simulink library "Energy_converter_Electrical_to_Mechanical"  (R2016a)
settings: Solver=ode1  StartTime=0.0  StopTime=Inf  FixedStep=0.001  RelTol=1e-3
undefined symbols (not defined in the file): API1dcac_efficiency, API2dcac_efficiency, API3dcac_efficiency, aux_power_state, AWR_InvStError, dat, DiscIntNeverNeededParam, EDCU_p_RefTqeMOT, emot_AcCmprFront_inertia, emot_AcCmprFront_nTab_3rdD, emot_AcCmprFront_pwrAC, emot_AcCmprFront_Tau, emot_AcCmprFront_trqTab_2ndD, emot_AcCmprFront_vltTab_1stD, emot_AcCmprRear_inertia, emot_AcCmprRear_nTab_3rdD, emot_AcCmprRear_pwrAC, emot_AcCmprRear_Tau, emot_AcCmprRear_trqTab_2ndD, emot_AcCmprRear_vltTab_1stD, emot_AirCmpr_inertia, emot_AirCmpr_nTab_3rdD, emot_AirCmpr_pwrAC, emot_AirCmpr_Tau, emot_AirCmpr_trqTab_2ndD, emot_AirCmpr_vltTab_1stD, emot_aircomp_power, emot_Cth_rotor, emot_Cth_stator, emot_dtrqEmotNeg, emot_dtrqEmotPtv, emot_inv_pwracTab_1st, emot_inv_pwrDC, emot_inv_pwrLoss, emot_inv_VrmsTab_2nd, emot_j, emot_mot_pwrLoss, emot_nTab_1stD, emot_pwrEtaTab_nRow, emot_pwrEtaTab_pwrTab, emot_pwrEtaTab_trqClm, emot_Rth_rotor_oil, emot_Rth_stator_oil, emot_Rth_stator_rotor, emot_tractiongroup, emot_Trotor_init, emot_trqMaxRow, emot_trqMinRow, emot_Tstator_init, emot_vltTab_3rdD, FirstDrivenAxleNoOfEmot, inv_Cth_cooling_plate, inv_Cth_diode, inv_Cth_IGBT, inv_n_IGBT_per_Switch, inv_Rth_cooling_plate_coolant, inv_Rth_PS_cooling_plate, inv_Tplate_init, inv_Tpowerstack_init, midAxleNoOfEmot ... (+6)
libraries: Electrical_converter x12, Energy_converter_Electrical_to_Mechanical x12, simulink x7
(part 6 of 8)

== system Energy_converter_Electrical_to_Mechanical/e-Motor/Thermic_Model_PMSM_slot2 ==
  P_WasteHeat_Rotor : Inport
  P_WasteHeat_Stator : Inport  Port=2
  T_Oil : Inport  Port=3
  T_Stator : Inport  Port=4
  T_Rotor : Inport  Port=5
  Add : Sum
  Add1 : Sum  Inputs=-+-
  Add2 : Sum  Inputs=++-
  C_Rotor : Subsystem
  C_Stator : Subsystem
  K2degC : Subsystem
  K2degC1 : Subsystem
  R_RotorOil : Subsystem
  R_StatorOil : Subsystem
  R_StatorRotor : Subsystem
  degC2K : Subsystem
  degC2K1 : Subsystem
  degC2K2 : Subsystem
  HeatFlow_eMotor_Oil : Outport
  T_Stator_new : Outport  Port=2
  T_Rotor_new : Outport  Port=3
  wires:
  C_Stator/1(T_new) -> K2degC/1(In1)
  C_Rotor/1(T_new) -> K2degC1/1(In1)
  Add/1 -> HeatFlow_eMotor_Oil/1
  R_StatorOil/1(dQ) -> Add1/1, Add/2
  [A] -> Add/1
  T_Stator/1 -> degC2K1/1(In1)
  P_WasteHeat_Stator/1 -> Add1/2
  Add1/1 -> C_Stator/1(P_Heat_eff)
  R_StatorRotor/1(dQ) -> Add2/1, Add1/3
  T_Rotor/1 -> degC2K2/1(In1)
  R_RotorOil/1(dQ) -> [A], Add2/3
  Add2/1 -> C_Rotor/1(P_Heat_eff)
  P_WasteHeat_Rotor/1 -> Add2/2
  K2degC/1(Out1) -> T_Stator_new/1
  K2degC1/1(Out1) -> T_Rotor_new/1
  T_Oil/1 -> degC2K/1(In1)  "T_Oil"
  degC2K/1(Out1) -> [B], R_StatorOil/1(T_Oil)
  degC2K1/1(Out1) -> R_StatorRotor/1(T_Stator), C_Stator/2(T), R_StatorOil/2(T_Stator)
  degC2K2/1(Out1) -> R_RotorOil/1(T_Rotor), C_Rotor/2(T), R_StatorRotor/2(T_Rotor)
  [B] -> R_RotorOil/2(T_Oil)

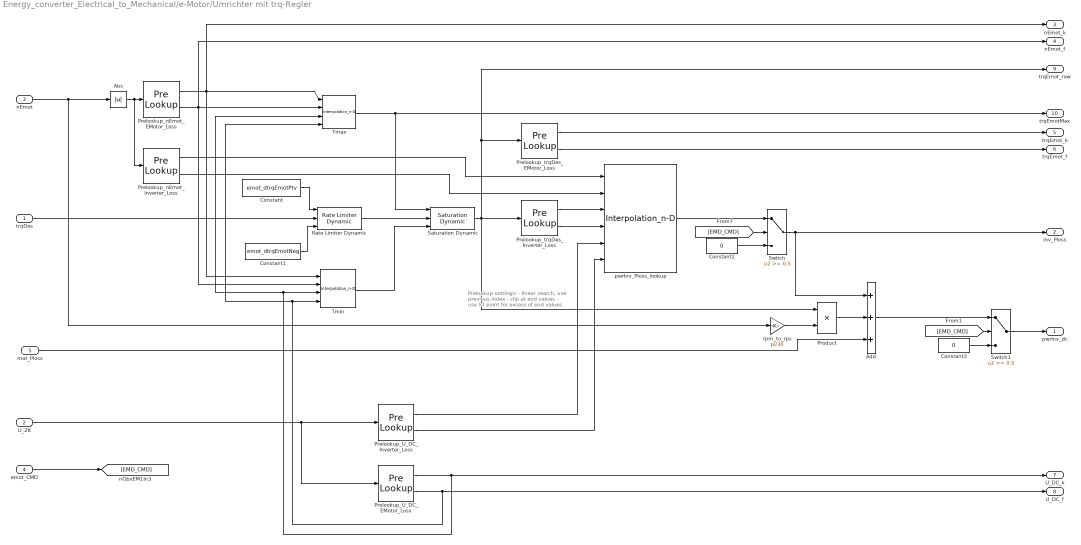
== system Energy_converter_Electrical_to_Mechanical/e-Motor/Umrichter mit trq-Regler ==
  note: Prelookup settings:
      | - linear search, use previous index
      | - clip at end values
      | - use lst point for
      | excess of end values
  trqDes : Inport
  U_ZK : Inport  Port=2
  nEmot : Inport  Port=3
  emot_CMD : Inport  Port=4
  mot_Ploss : Inport  Port=5
  Abs : Abs
  Add : Sum  Inputs=+++
  Constant : Constant  Value=emot_dtrqEmotPtv
  Constant1 : Constant  Value=emot_dtrqEmotNeg
  Constant2 : Constant  Value=0
  Constant3 : Constant  Value=0
  Prelookup_U_DC_EMotor_Loss : PreLookup  BreakpointsData=emot_vltTab_3rdD  IndexSearchMethod=Linear search  BeginIndexSearchUsingPreviousIndexResult=on  UseLastBreakpoint=on
  Prelookup_U_DC_Inverter_Loss : PreLookup  BreakpointsData=inv_vltTab_3rdD  IndexSearchMethod=Linear search  BeginIndexSearchUsingPreviousIndexResult=on  UseLastBreakpoint=on
  Prelookup_nEmot_EMotor_Loss : PreLookup  BreakpointsData=emot_nTab_1stD  IndexSearchMethod=Linear search  BeginIndexSearchUsingPreviousIndexResult=on  UseLastBreakpoint=on
  Prelookup_nEmot_Inverter_Loss : PreLookup  BreakpointsData=inv_nTab_1stD  IndexSearchMethod=Linear search  BeginIndexSearchUsingPreviousIndexResult=on  UseLastBreakpoint=on
  Prelookup_trqDes_EMotor_Loss : PreLookup  BreakpointsData=emot_trqTab_2ndD  IndexSearchMethod=Linear search  BeginIndexSearchUsingPreviousIndexResult=on  UseLastBreakpoint=on
  Prelookup_trqDes_Inverter_Loss : PreLookup  BreakpointsData=inv_trqTab_2ndD  IndexSearchMethod=Linear search  BeginIndexSearchUsingPreviousIndexResult=on  UseLastBreakpoint=on
  Product : Product  RndMeth=Zero
  Rate Limiter Dynamic : simulink/Discontinuities/Rate Limiter Dynamic
  Saturation Dynamic : simulink/Discontinuities/Saturation Dynamic  OutMin=[]  OutMax=[]  OutDataTypeStr=Inherit: Same as second input  OutDataType=fixdt(1, 16)  OutScaling=2^-10  DoSatur=off
  Switch : Switch  Threshold=0.5
  Switch1 : Switch  Threshold=0.5
  Tmax : Interpolation_n-D  Table=emot_trqMaxRow  ExtrapMethod=Clip  ValidIndexMayReachLast=on
  Tmin : Interpolation_n-D  Table=emot_trqMinRow  ExtrapMethod=Clip  ValidIndexMayReachLast=on
  pwrInv_Ploss_lookup : Interpolation_n-D  NumberOfTableDimensions=3  Table=emot_inv_pwrLoss  ExtrapMethod=Clip  ValidIndexMayReachLast=on
      settings: InputPortMap=u0,u1,u2,u3,u4,u5
  rpm_to_rps : Gain  Gain=pi/30
  pwrInv_dc : Outport
  inv_Ploss : Outport  Port=2
  nEmot_k : Outport  Port=3
  nEmot_f : Outport  Port=4
  trqEmot_k : Outport  Port=5
  trqEmot_f : Outport  Port=6
  U_DC_k : Outport  Port=7
  U_DC_f : Outport  Port=8
  trqEmot_raw : Outport  Port=9
  trqEmotMax : Outport  Port=10
  wires:
  Prelookup_trqDes_Inverter_Loss/2 -> pwrInv_Ploss_lookup/4
  Prelookup_trqDes_Inverter_Loss/1 -> pwrInv_Ploss_lookup/3
  Switch/1 -> Add/1, inv_Ploss/1
  Saturation Dynamic/1 -> trqEmot_raw/1, Prelookup_trqDes_EMotor_Loss/1, Product/1, Prelookup_trqDes_Inverter_Loss/1
  Product/1 -> Add/2
  rpm_to_rps/1 -> Product/2
  mot_Ploss/1 -> Add/3
  Constant3/1 -> Switch1/3
  [EMD_CMD] -> Switch1/2
  Add/1 -> Switch1/1
  Constant2/1 -> Switch/3
  [EMD_CMD] -> Switch/2
  emot_CMD/1 -> [EMD_CMD]
  pwrInv_Ploss_lookup/1 -> Switch/1
  Switch1/1 -> pwrInv_dc/1
  Rate Limiter Dynamic/1 -> Saturation Dynamic/2
  Constant1/1 -> Rate Limiter Dynamic/3
  Constant/1 -> Rate Limiter Dynamic/1
  nEmot/1 -> Abs/1, rpm_to_rps/1
  Tmax/1 -> Saturation Dynamic/1, trqEmotMax/1
  Tmin/1 -> Saturation Dynamic/3
  U_ZK/1 -> Prelookup_U_DC_EMotor_Loss/1, Prelookup_U_DC_Inverter_Loss/1
  Prelookup_U_DC_Inverter_Loss/2 -> pwrInv_Ploss_lookup/6
  Prelookup_U_DC_Inverter_Loss/1 -> pwrInv_Ploss_lookup/5
  Prelookup_nEmot_EMotor_Loss/2 -> nEmot_f/1, Tmax/2, Tmin/2
  Prelookup_nEmot_EMotor_Loss/1 -> nEmot_k/1, Tmin/1, Tmax/1
  trqDes/1 -> Rate Limiter Dynamic/2
  Abs/1 -> Prelookup_nEmot_EMotor_Loss/1, Prelookup_nEmot_Inverter_Loss/1
  Prelookup_trqDes_EMotor_Loss/1 -> trqEmot_k/1
  Prelookup_trqDes_EMotor_Loss/2 -> trqEmot_f/1
  Prelookup_U_DC_EMotor_Loss/1 -> Tmin/3, Tmax/3, U_DC_k/1
  Prelookup_U_DC_EMotor_Loss/2 -> U_DC_f/1, Tmin/4, Tmax/4
  Prelookup_nEmot_Inverter_Loss/1 -> pwrInv_Ploss_lookup/1
  Prelookup_nEmot_Inverter_Loss/2 -> pwrInv_Ploss_lookup/2

== system Energy_converter_Electrical_to_Mechanical/e-Motor/updatePortNames ==

== system Energy_converter_Electrical_to_Mechanical/e-Motor_Gen2/Fahrmotoren ==
  nEmot_k : Inport
  nEmot_f : Inport  Port=2
  trqEmot_k : Inport  Port=3
  trqEmot_f : Inport  Port=4
  U_DC_k : Inport  Port=5
  U_DC_f : Inport  Port=6
  mot_Ploss_lookup : Interpolation_n-D  NumberOfTableDimensions=3  Table=emot_mot_pwrLoss  ExtrapMethod=Clip  ValidIndexMayReachLast=on
      settings: InputPortMap=u0,u1,u2,u3,u4,u5
  mot_Ploss : Outport
  wires:
  mot_Ploss_lookup/1 -> mot_Ploss/1
  nEmot_f/1 -> mot_Ploss_lookup/2
  nEmot_k/1 -> mot_Ploss_lookup/1
  trqEmot_k/1 -> mot_Ploss_lookup/3
  trqEmot_f/1 -> mot_Ploss_lookup/4
  U_DC_k/1 -> mot_Ploss_lookup/5
  U_DC_f/1 -> mot_Ploss_lookup/6

== system Energy_converter_Electrical_to_Mechanical/e-Motor_Gen2/Thermic_Model_Inverter ==
  P_WasteHeat_Powerstack : Inport
  T_Coolant : Inport  Port=2
  T_Powerstack : Inport  Port=3
  T_Plate : Inport  Port=4
  Add : Sum  Inputs=+-
  Add1 : Sum  Inputs=+-
  C_IGBT_and_Diode : Subsystem
  C_Plate : Subsystem
  Gain : Gain  Gain=1/inv_n_IGBT_per_Switch
  Gain2 : Gain  Gain=inv_n_IGBT_per_Switch
  R_PS-Plate : Subsystem
  R_Plate-Coolant : Subsystem
  P_Coolant : Outport
  T_Powerstack_new : Outport  Port=2
  T_Plate_new : Outport  Port=3
  wires:
  Add/1 -> C_IGBT_and_Diode/1(P_Heat_eff)
  P_WasteHeat_Powerstack/1 -> Gain/1
  Add1/1 -> C_Plate/1(P_Heat_eff)
  T_Powerstack/1 -> R_PS-Plate/1(T_IGBT), C_IGBT_and_Diode/2(T)
  C_IGBT_and_Diode/1(T_new) -> T_Powerstack_new/1
  T_Plate/1 -> R_Plate-Coolant/1(T_Plate), R_PS-Plate/2(T_Plate), C_Plate/2(T)
  C_Plate/1(T_new) -> T_Plate_new/1
  T_Coolant/1 -> R_Plate-Coolant/2(T_Coolant)
  Gain/1 -> Add/1
  Gain2/1 -> P_Coolant/1
  R_PS-Plate/1(dQ) -> Add/2, Add1/1
  R_Plate-Coolant/1(dQ) -> Add1/2, Gain2/1

== system Energy_converter_Electrical_to_Mechanical/e-Motor_Gen2/Thermic_Model_PMSM_slot2 ==
  P_WasteHeat_Rotor : Inport
  P_WasteHeat_Stator : Inport  Port=2
  T_Oil : Inport  Port=3
  T_Stator : Inport  Port=4
  T_Rotor : Inport  Port=5
  Add : Sum
  Add1 : Sum  Inputs=-+-
  Add2 : Sum  Inputs=++-
  C_Rotor : Subsystem
  C_Stator : Subsystem
  K2degC : Subsystem
  K2degC1 : Subsystem
  R_RotorOil : Subsystem
  R_StatorOil : Subsystem
  R_StatorRotor : Subsystem
  degC2K : Subsystem
  degC2K1 : Subsystem
  degC2K2 : Subsystem
  HeatFlow_eMotor_Oil : Outport
  T_Stator_new : Outport  Port=2
  T_Rotor_new : Outport  Port=3
  wires:
  C_Stator/1(T_new) -> K2degC/1(In1)
  C_Rotor/1(T_new) -> K2degC1/1(In1)
  Add/1 -> HeatFlow_eMotor_Oil/1
  R_StatorOil/1(dQ) -> Add1/1, Add/2
  [A] -> Add/1
  T_Stator/1 -> degC2K1/1(In1)
  P_WasteHeat_Stator/1 -> Add1/2
  Add1/1 -> C_Stator/1(P_Heat_eff)
  R_StatorRotor/1(dQ) -> Add2/1, Add1/3
  T_Rotor/1 -> degC2K2/1(In1)
  R_RotorOil/1(dQ) -> [A], Add2/3
  Add2/1 -> C_Rotor/1(P_Heat_eff)
  P_WasteHeat_Rotor/1 -> Add2/2
  K2degC/1(Out1) -> T_Stator_new/1
  K2degC1/1(Out1) -> T_Rotor_new/1
  T_Oil/1 -> degC2K/1(In1)  "T_Oil"
  degC2K/1(Out1) -> [B], R_StatorOil/1(T_Oil)
  degC2K1/1(Out1) -> R_StatorRotor/1(T_Stator), C_Stator/2(T), R_StatorOil/2(T_Stator)
  degC2K2/1(Out1) -> R_RotorOil/1(T_Rotor), C_Rotor/2(T), R_StatorRotor/2(T_Rotor)
  [B] -> R_RotorOil/2(T_Oil)

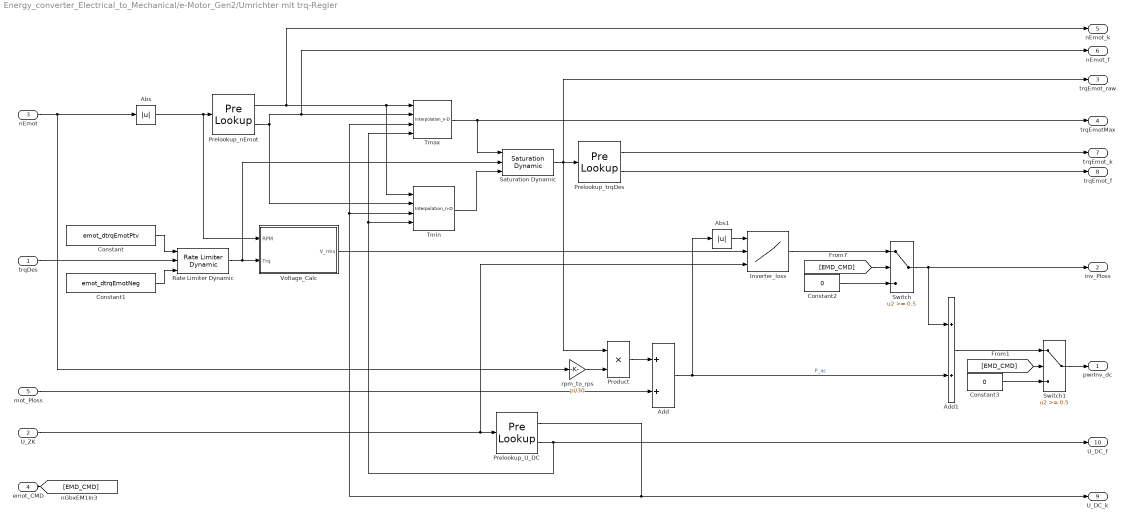
== system Energy_converter_Electrical_to_Mechanical/e-Motor_Gen2/Umrichter mit trq-Regler ==
  trqDes : Inport
  U_ZK : Inport  Port=2
  nEmot : Inport  Port=3
  emot_CMD : Inport  Port=4
  mot_Ploss : Inport  Port=5
  Abs : Abs
  Abs1 : Abs
  Add : Sum
  Add1 : Sum
  Constant : Constant  Value=emot_dtrqEmotPtv
  Constant1 : Constant  Value=emot_dtrqEmotNeg
  Constant2 : Constant  Value=0
  Constant3 : Constant  Value=0
  Inverter_loss : Lookup_n-D  NumberOfTableDimensions=3  BreakpointsForDimension1=emot_inv_pwracTab_1st  BreakpointsForDimension2=emot_inv_VrmsTab_2nd  BreakpointsForDimension3=emot_vltTab_3rdD  Table=emot_inv_pwrLoss  ExtrapMethod=Clip  UseLastTableValue=on  RndMeth=Simplest  InputSameDT=on
  Prelookup_U_DC : PreLookup  BreakpointsData=emot_vltTab_3rdD  IndexSearchMethod=Linear search  BeginIndexSearchUsingPreviousIndexResult=on  UseLastBreakpoint=on
  Prelookup_nEmot : PreLookup  BreakpointsData=emot_nTab_1stD  IndexSearchMethod=Linear search  BeginIndexSearchUsingPreviousIndexResult=on  UseLastBreakpoint=on
  Prelookup_trqDes : PreLookup  BreakpointsData=drvemot_trqTab_2ndD  IndexSearchMethod=Linear search  BeginIndexSearchUsingPreviousIndexResult=on  UseLastBreakpoint=on
  Product : Product  RndMeth=Zero
  Rate Limiter Dynamic : simulink/Discontinuities/Rate Limiter Dynamic
  Saturation Dynamic : simulink/Discontinuities/Saturation Dynamic  OutMin=[]  OutMax=[]  OutDataTypeStr=Inherit: Same as second input  OutDataType=fixdt(1, 16)  OutScaling=2^-10  DoSatur=off
  Switch : Switch  Threshold=0.5
  Switch1 : Switch  Threshold=0.5
  Tmax : Interpolation_n-D  Table=emot_trqMaxRow  ExtrapMethod=Clip  ValidIndexMayReachLast=on
  Tmin : Interpolation_n-D  Table=emot_trqMinRow  ExtrapMethod=Clip  ValidIndexMayReachLast=on
  Voltage_Calc : Subsystem
  rpm_to_rps : Gain  Gain=pi/30
  pwrInv_dc : Outport
  inv_Ploss : Outport  Port=2
  trqEmot_raw : Outport  Port=3
  trqEmotMax : Outport  Port=4
  nEmot_k : Outport  Port=5
  nEmot_f : Outport  Port=6
  trqEmot_k : Outport  Port=7
  trqEmot_f : Outport  Port=8
  U_DC_k : Outport  Port=9
  U_DC_f : Outport  Port=10
  wires:
  Abs1/1 -> Inverter_loss/1
  Add/1 -> Abs1/1, Add1/2  "P_ac"
  Switch/1 -> Add1/1, inv_Ploss/1
  mot_Ploss/1 -> Add/2
  U_ZK/1 -> Inverter_loss/3, Prelookup_U_DC/1
  Product/1 -> Add/1
  rpm_to_rps/1 -> Product/2
  Constant3/1 -> Switch1/3
  [EMD_CMD] -> Switch1/2
  Add1/1 -> Switch1/1
  Constant2/1 -> Switch/3
  [EMD_CMD] -> Switch/2
  emot_CMD/1 -> [EMD_CMD]
  Inverter_loss/1 -> Switch/1
  Saturation Dynamic/1 -> Product/1, trqEmot_raw/1, Prelookup_trqDes/1
  Switch1/1 -> pwrInv_dc/1
  Rate Limiter Dynamic/1 -> Saturation Dynamic/2, Voltage_Calc/2(Trq)
  Constant1/1 -> Rate Limiter Dynamic/3
  Constant/1 -> Rate Limiter Dynamic/1
  nEmot/1 -> rpm_to_rps/1, Abs/1
  Tmax/1 -> trqEmotMax/1, Saturation Dynamic/1
  Tmin/1 -> Saturation Dynamic/3
  Prelookup_trqDes/1 -> trqEmot_k/1
  Prelookup_trqDes/2 -> trqEmot_f/1
  Prelookup_U_DC/2 -> Tmax/4, Tmin/4, U_DC_f/1
  Prelookup_U_DC/1 -> U_DC_k/1, Tmax/3, Tmin/3
  Prelookup_nEmot/2 -> Tmin/2, nEmot_f/1, Tmax/2
  Prelookup_nEmot/1 -> nEmot_k/1, Tmax/1, Tmin/1
  trqDes/1 -> Rate Limiter Dynamic/2
  Abs/1 -> Voltage_Calc/1(RPM), Prelookup_nEmot/1
  Voltage_Calc/1(V_rms) -> Inverter_loss/2

== system Energy_converter_Electrical_to_Mechanical/e-Motor_Gen2/updatePortNames ==

== system Energy_converter_Electrical_to_Mechanical/e-Motor_chy_proposal/Fahrmotoren ==
  nEmot_k : Inport
  nEmot_f : Inport  Port=2
  trqEmot_k : Inport  Port=3
  trqEmot_f : Inport  Port=4
  U_DC_k : Inport  Port=5
  U_DC_f : Inport  Port=6
  mot_Ploss_lookup : Interpolation_n-D  NumberOfTableDimensions=3  Table=emot_mot_pwrLoss  ExtrapMethod=Clip  ValidIndexMayReachLast=on
      settings: InputPortMap=u0,u1,u2,u3,u4,u5
  mot_Ploss : Outport
  wires:
  mot_Ploss_lookup/1 -> mot_Ploss/1
  nEmot_f/1 -> mot_Ploss_lookup/2
  nEmot_k/1 -> mot_Ploss_lookup/1
  trqEmot_k/1 -> mot_Ploss_lookup/3
  trqEmot_f/1 -> mot_Ploss_lookup/4
  U_DC_k/1 -> mot_Ploss_lookup/5
  U_DC_f/1 -> mot_Ploss_lookup/6

== system Energy_converter_Electrical_to_Mechanical/e-Motor_chy_proposal/Umrichter mit trq-Regler ==
  note: cyan blocks: adapted to compact hybrid
  note: To be decided: Is this block necessary at all?
  note: Prelookup settings:
      | - linear search, use previous index
      | - clip at end values
      | - use lst point for
      | excess of end values
  trqDes : Inport
  U_ZK : Inport  Port=2
  nEmot : Inport  Port=3
  Abs : Abs
  Constant : Constant  Value=emot_dtrqEmotPtv
  Constant1 : Constant  Value=emot_dtrqEmotNeg
  Gain : Gain  Gain=1/60
  Gain1 : Gain
  Gain2 : Gain
  Gain3 : Gain
  Memory : Memory
  Prelookup_U_DC : PreLookup  BreakpointsData=emot_vltTab_3rdD  IndexSearchMethod=Linear search  BeginIndexSearchUsingPreviousIndexResult=on  UseLastBreakpoint=on
  Prelookup_nEmot : PreLookup  BreakpointsData=emot_nTab_1stD  IndexSearchMethod=Linear search  BeginIndexSearchUsingPreviousIndexResult=on  UseLastBreakpoint=on
  Prelookup_trqDes : PreLookup  BreakpointsData=emot_trqTab_2ndD  IndexSearchMethod=Linear search  BeginIndexSearchUsingPreviousIndexResult=on  UseLastBreakpoint=on
  Rate Limiter Dynamic : Subsystem  mask(Rate Limiter Dynamic){}
      mask help: Simulink:masks:RateLimiterDynamic_MD
      mask Display: plot([0.15 0.95],[.5 .5],[.5 .5],[0.05 0.95],0.05+0.9*[.2 .8],0.05+0.9*[0 1]);
  Saturation Dynamic : Subsystem  mask(Saturation Dynamic){OutMin=[], OutMax=[], OutDataTypeStr=Inherit: Same as second input, OutputDataTypeScalingMode=Same as second input, OutDataType=fixdt(1, 16), OutScaling=2^-10, LockScale=off, RndMeth=Floor, DoSatur=off}
      mask prompts: OutMin "Simulink:masks:OutputMinimum_MP"; OutMax "Simulink:masks:OutputMaximum_MP"; OutDataTypeStr "Simulink:masks:OutputDataType_MP"; OutputDataTypeScalingMode "Simulink:masks:OutputDataTypeMode_MP"; OutDataType "Simulink:masks:OutputDataTypeegFixdt116Fixdtsingle_MP"; OutScaling "Simulink:masks:OutputScalingSlopeEg29OrSlopeBias_MP"; LockScale "Simulink:masks:LockOutputDataTypeAgainstFxpTools_MP"; RndMeth "Simulink:masks:IntegerRoundingMode_MP"; DoSatur "Simulink:masks:SaturateOnIntegerOverflow_MP"
      mask help: Simulink:masks:SaturationDynamic_MD
      mask init:
      | blkH = gcbh;
      | blkName = getfullname(blkH);
      | 
      | switch_blks = {'Switch','Switch2'}; 
      | for i = 1:length(switch_blks)
      |   set_param([blkName,'/',switch_blks{i}], ...
      |       'RndMeth', RndMeth, ...
      | 	  'DoSatur', DoSatur);
      | end
      | 
      | propBlk = [blkName, '/Data Type Propagation'];
      | 
      | if strcmp(OutputDataTypeScalingMode, 'Same as second input')
      |     set_param(propBlk, 'PropDataTypeMode', 'Inherit via propagation rule', ...
      |                        'PropScalingMode',  'Inherit via propagation rule');
      | else
      |     scaling = OutScaling;
      |     scalingMode = 'Specify via dialog';
      |     switch OutputDataTypeScalingMode
      |       case 'double'
      |         dataType = 'fixdt(''double'')';
      |       case 'single'
      |         dataType = 'fixdt(''single'')';
      |       case 'int8'
      |         dataType = 'fixdt(1,8,0)';
      |       case 'uint8'
      |         dataType = 'fixdt(0,8,0)';
      |       case 'int16'
      |         dataType = 'fixdt(1,16,0)';
      |       case 'uint16'
      |         dataType = 'fixdt(0,16,0)';
      |       case 'int32'
      |         dataType = 'fixdt(1,32,0)';
      |       case 'uint32'
      |         dataType = 'fixdt(0,32,0)';
      |       case 'Specify via dialog'
      |         dataType = OutDataType;
      |         if ~isempty(OutDataTypeStr) && isa(OutDataTypeStr,'Simulink.NumericType') 
      |           if strcmp(OutDataTypeStr.DataTypeMode, 'Fixed-point: unspecified scaling') 
      |             scalingMode = 'Obtain via best precision';
      |             range = [OutMin OutMax];
      |             range = range(~isinf(range));
      |             set_param(propBlk, 'ValuesUsedBestPrec', mat2str(range));
      |           end
      |         end
      |     end
      |     
      |     set_param(propBlk, 'PropDataTypeMode', 'Specify via dialog', ...
      |                        'PropScalingMode',  scalingMode, ...
      |                        'PropDataType',     dataType, ...
      |                        'PropScaling',      scaling);
      | end
      mask Callback OutDataTypeStr: fixptdialog(gcbh)
      mask TypeOptions OutputDataTypeScalingMode: double | single | int8 | uint8 | int16 | uint16 | int32 | uint32 | Specify via dialog | Same as second input
      mask Callback OutputDataTypeScalingMode: fixptdialog(gcbh)
      mask Callback OutDataType: fixptdialog(gcbh)
      mask TypeOptions RndMeth: Simulink:masks:Ceiling | Simulink:masks:Convergent | Simulink:masks:Floor | Simulink:masks:Nearest | Simulink:masks:Round | Simulink:masks:Simplest | Simulink:masks:Zero
      mask Display: plot([0.15 0.85],[.5 .5],[.5 .5],[0.05 0.95],0.15+0.7*[0 .25 .75 1],0.05+0.9*[.25 .25 .75 .75]);
  Tmax : Interpolation_n-D  Table=emot_trqMaxRow  ExtrapMethod=Clip  ValidIndexMayReachLast=on
  Tmin : Interpolation_n-D  Table=emot_trqMinRow  ExtrapMethod=Clip  ValidIndexMayReachLast=on
  Transfer Fcn : TransferFcn  Denominator=1
  Umrechnung in el Leistung [W] : Subsystem
  Umrechnung in el Leistung [W]_Max : Subsystem
  const : Constant
  pwrInv_DC_lookup : Interpolation_n-D  NumberOfTableDimensions=3  Table=emot_inv_pwrDC  ExtrapMethod=Clip  ValidIndexMayReachLast=on
      settings: InputPortMap=u0,u1,u2,u3,u4,u5
  pwrInv_Ploss_lookup : Interpolation_n-D  NumberOfTableDimensions=3  Table=emot_inv_pwrLoss  ExtrapMethod=Clip  ValidIndexMayReachLast=on
      settings: InputPortMap=u0,u1,u2,u3,u4,u5
  switch : Switch  Threshold=0.5  SaturateOnIntegerOverflow=on  InputSameDT=on
      settings: AttributesFormatString=<threshold=%<threshold>>
  pwrInv_dc : Outport
  inv_Ploss : Outport  Port=2
  nEmot_k : Outport  Port=3
  nEmot_f : Outport  Port=4
  trqEmot_k : Outport  Port=5
  trqEmot_f : Outport  Port=6
  U_DC_k : Outport  Port=7
  U_DC_f : Outport  Port=8
  trqEmot_raw : Outport  Port=9
  trqEmotMax : Outport  Port=10
  pwrInvmax : Outport  Port=11
  wires:
  Abs/1 -> Prelookup_nEmot/1
  Umrechnung in el Leistung [W]_Max/1(pwrTdc) -> pwrInvmax/1
  Gain3/1 -> switch/1
  Gain2/1 -> inv_Ploss/1
  Gain1/1 -> Prelookup_trqDes/1
  const/1 -> switch/2
  Umrechnung in el Leistung [W]/1(pwrTdc) -> switch/3
  pwrInv_DC_lookup/1 -> Gain3/1
  switch/1 -> pwrInv_dc/1
  Gain/1 -> Umrechnung in el Leistung [W]/2(nEmot)
  trqDes/1 -> Memory/1
  Transfer Fcn/1 -> Rate Limiter Dynamic/2(u)
  Rate Limiter Dynamic/1(Y) -> Saturation Dynamic/2(u)
  Constant1/1 -> Rate Limiter Dynamic/3(lo)
  Constant/1 -> Rate Limiter Dynamic/1(up)
  nEmot/1 -> Gain/1, Umrechnung in el Leistung [W]_Max/2(nEmot), Abs/1
  Tmax/1 -> trqEmotMax/1, Umrechnung in el Leistung [W]_Max/1(trqEmot), Saturation Dynamic/1(up)
  Tmin/1 -> Saturation Dynamic/3(lo)
  U_ZK/1 -> Prelookup_U_DC/1
  Saturation Dynamic/1(y) -> Umrechnung in el Leistung [W]/1(trqEmot), Gain1/1, trqEmot_raw/1
  Prelookup_trqDes/1 -> trqEmot_k/1, pwrInv_DC_lookup/3, pwrInv_Ploss_lookup/3
  Prelookup_trqDes/2 -> trqEmot_f/1, pwrInv_DC_lookup/4, pwrInv_Ploss_lookup/4
  Prelookup_U_DC/2 -> Tmin/2, Tmax/2, U_DC_f/1, pwrInv_Ploss_lookup/6, pwrInv_DC_lookup/6
  Prelookup_U_DC/1 -> Tmax/1, Tmin/1, pwrInv_Ploss_lookup/5, U_DC_k/1, pwrInv_DC_lookup/5
  pwrInv_Ploss_lookup/1 -> Gain2/1
  Prelookup_nEmot/2 -> Tmin/4, nEmot_f/1, Tmax/4, pwrInv_DC_lookup/2, pwrInv_Ploss_lookup/2
  Prelookup_nEmot/1 -> Tmin/3, nEmot_k/1, Tmax/3, pwrInv_DC_lookup/1, pwrInv_Ploss_lookup/1
  Memory/1 -> Transfer Fcn/1

== system Energy_converter_Electrical_to_Mechanical/e-Motor_chy_proposal/updatePortNames ==

== system Energy_converter_Electrical_to_Mechanical/AWR_DriveEmot/AWR 1 TX/Nm_to_percent ==
  Nm_Torque : Inport
  Reference_Torque : Inport  Port=2
  Constant : Constant  Value=100
  Divide1 : Product  Inputs=*/
  Product1 : Product  RndMeth=Zero
  Torque_Percentage : Outport
  wires:
  Constant/1 -> Product1/2
  Divide1/1 -> Product1/1
  Reference_Torque/1 -> Divide1/2  "Reference_Torque"
  Product1/1 -> Torque_Percentage/1  "Torque_Percentage"
  Nm_Torque/1 -> Divide1/1  "Nm_Torque"

== system Energy_converter_Electrical_to_Mechanical/AWR_DriveEmot/AWR 1 TX/Nm_to_percent1 ==
  Nm_Torque : Inport
  Reference_Torque : Inport  Port=2
  Constant : Constant  Value=100
  Divide1 : Product  Inputs=*/
  Product1 : Product  RndMeth=Zero
  Torque_Percentage : Outport
  wires:
  Nm_Torque/1 -> Divide1/1  "Nm_Torque"
  Product1/1 -> Torque_Percentage/1  "Torque_Percentage"
  Reference_Torque/1 -> Divide1/2  "Reference_Torque"
  Divide1/1 -> Product1/1
  Constant/1 -> Product1/2

== system Energy_converter_Electrical_to_Mechanical/AWR_DriveEmot/AWR 1 TX/Nm_to_percent2 ==
  Nm_Torque : Inport
  Reference_Torque : Inport  Port=2
  Constant : Constant  Value=100
  Divide1 : Product  Inputs=*/
  Product1 : Product  RndMeth=Zero
  Torque_Percentage : Outport
  wires:
  Constant/1 -> Product1/2
  Divide1/1 -> Product1/1
  Reference_Torque/1 -> Divide1/2  "Reference_Torque"
  Product1/1 -> Torque_Percentage/1  "Torque_Percentage"
  Nm_Torque/1 -> Divide1/1  "Nm_Torque"

== system Energy_converter_Electrical_to_Mechanical/AWR_DriveEmot/AWR 2 TX/Nm_to_percent ==
  Nm_Torque : Inport
  Reference_Torque : Inport  Port=2
  Constant : Constant  Value=100
  Divide1 : Product  Inputs=*/
  Product1 : Product  RndMeth=Zero
  Torque_Percentage : Outport
  wires:
  Constant/1 -> Product1/2
  Divide1/1 -> Product1/1
  Reference_Torque/1 -> Divide1/2  "Reference_Torque"
  Product1/1 -> Torque_Percentage/1  "Torque_Percentage"
  Nm_Torque/1 -> Divide1/1  "Nm_Torque"

== system Energy_converter_Electrical_to_Mechanical/AWR_DriveEmot/AWR 2 TX/Nm_to_percent1 ==
  Nm_Torque : Inport
  Reference_Torque : Inport  Port=2
  Constant : Constant  Value=100
  Divide1 : Product  Inputs=*/
  Product1 : Product  RndMeth=Zero
  Torque_Percentage : Outport
  wires:
  Nm_Torque/1 -> Divide1/1  "Nm_Torque"
  Product1/1 -> Torque_Percentage/1  "Torque_Percentage"
  Reference_Torque/1 -> Divide1/2  "Reference_Torque"
  Divide1/1 -> Product1/1
  Constant/1 -> Product1/2

== system Energy_converter_Electrical_to_Mechanical/AWR_DriveEmot/AWR 2 TX/Nm_to_percent2 ==
  Nm_Torque : Inport
  Reference_Torque : Inport  Port=2
  Constant : Constant  Value=100
  Divide1 : Product  Inputs=*/
  Product1 : Product  RndMeth=Zero
  Torque_Percentage : Outport
  wires:
  Constant/1 -> Product1/2
  Divide1/1 -> Product1/1
  Reference_Torque/1 -> Divide1/2  "Reference_Torque"
  Product1/1 -> Torque_Percentage/1  "Torque_Percentage"
  Nm_Torque/1 -> Divide1/1  "Nm_Torque"

== system Energy_converter_Electrical_to_Mechanical/AWR_DriveEmot/AWR 3 TX/Nm_to_percent ==
  Nm_Torque : Inport
  Reference_Torque : Inport  Port=2
  Constant : Constant  Value=100
  Divide1 : Product  Inputs=*/
  Product1 : Product  RndMeth=Zero
  Torque_Percentage : Outport
  wires:
  Nm_Torque/1 -> Divide1/1  "Nm_Torque"
  Product1/1 -> Torque_Percentage/1  "Torque_Percentage"
  Reference_Torque/1 -> Divide1/2  "Reference_Torque"
  Divide1/1 -> Product1/1
  Constant/1 -> Product1/2

== system Energy_converter_Electrical_to_Mechanical/AWR_DriveEmot/AWR 3 TX/Nm_to_percent1 ==
  Nm_Torque : Inport
  Reference_Torque : Inport  Port=2
  Constant : Constant  Value=100
  Divide1 : Product  Inputs=*/
  Product1 : Product  RndMeth=Zero
  Torque_Percentage : Outport
  wires:
  Constant/1 -> Product1/2
  Divide1/1 -> Product1/1
  Reference_Torque/1 -> Divide1/2  "Reference_Torque"
  Product1/1 -> Torque_Percentage/1  "Torque_Percentage"
  Nm_Torque/1 -> Divide1/1  "Nm_Torque"

== system Energy_converter_Electrical_to_Mechanical/AWR_DriveEmot/AWR 3 TX/Nm_to_percent2 ==
  Nm_Torque : Inport
  Reference_Torque : Inport  Port=2
  Constant : Constant  Value=100
  Divide1 : Product  Inputs=*/
  Product1 : Product  RndMeth=Zero
  Torque_Percentage : Outport
  wires:
  Nm_Torque/1 -> Divide1/1  "Nm_Torque"
  Product1/1 -> Torque_Percentage/1  "Torque_Percentage"
  Reference_Torque/1 -> Divide1/2  "Reference_Torque"
  Divide1/1 -> Product1/1
  Constant/1 -> Product1/2

== system Energy_converter_Electrical_to_Mechanical/AWR_DriveEmot/AWR 4 TX/Nm_to_percent ==
  Nm_Torque : Inport
  Reference_Torque : Inport  Port=2
  Constant : Constant  Value=100
  Divide1 : Product  Inputs=*/
  Product1 : Product  RndMeth=Zero
  Torque_Percentage : Outport
  wires:
  Constant/1 -> Product1/2
  Divide1/1 -> Product1/1
  Reference_Torque/1 -> Divide1/2  "Reference_Torque"
  Product1/1 -> Torque_Percentage/1  "Torque_Percentage"
  Nm_Torque/1 -> Divide1/1  "Nm_Torque"

== system Energy_converter_Electrical_to_Mechanical/AWR_DriveEmot/AWR 4 TX/Nm_to_percent1 ==
  Nm_Torque : Inport
  Reference_Torque : Inport  Port=2
  Constant : Constant  Value=100
  Divide1 : Product  Inputs=*/
  Product1 : Product  RndMeth=Zero
  Torque_Percentage : Outport
  wires:
  Nm_Torque/1 -> Divide1/1  "Nm_Torque"
  Product1/1 -> Torque_Percentage/1  "Torque_Percentage"
  Reference_Torque/1 -> Divide1/2  "Reference_Torque"
  Divide1/1 -> Product1/1
  Constant/1 -> Product1/2

== system Energy_converter_Electrical_to_Mechanical/AWR_DriveEmot/AWR 4 TX/Nm_to_percent2 ==
  Nm_Torque : Inport
  Reference_Torque : Inport  Port=2
  Constant : Constant  Value=100
  Divide1 : Product  Inputs=*/
  Product1 : Product  RndMeth=Zero
  Torque_Percentage : Outport
  wires:
  Constant/1 -> Product1/2
  Divide1/1 -> Product1/1
  Reference_Torque/1 -> Divide1/2  "Reference_Torque"
  Product1/1 -> Torque_Percentage/1  "Torque_Percentage"
  Nm_Torque/1 -> Divide1/1  "Nm_Torque"

== system Energy_converter_Electrical_to_Mechanical/AWR_DriveEmot/AWR1_4/ZeroWhenNotReady1 ==
  Bus Creator4 : BusCreator  Inputs=11
  zero_EMD1_ACT_DcLinkPower : Constant  Value=0
  zero_EMD1_ACT_DcLinkVoltage : Constant  Value=0
  zero_EMD1_ACT_DigitalInput1 : Constant  Value=0
  zero_EMD1_ACT_InverterState : Constant  Value=0
  zero_EMD1_ACT_MaxJunctionTemperature : Constant  Value=0
  zero_EMD1_ACT_MaximumAvailableTorque : Constant  Value=0
  zero_EMD1_ACT_MotorSpeed : Constant  Value=0
  zero_EMD1_ACT_MotorTemperature : Constant  Value=0
  zero_EMD1_ACT_MotorTorque : Constant  Value=0
  zero_EMD1_ACT_ReferenceTorqueLimited : Constant  Value=0
  zero_trqEmot1DesPhy : Constant  Value=0
  Out1 : Outport
  wires:
  zero_EMD1_ACT_MotorTemperature/1 -> Bus Creator4/11  "EMD_ACT_MotorTemperature"
  zero_EMD1_ACT_MaxJunctionTemperature/1 -> Bus Creator4/10  "EMD_ACT_MaxJunctionTemperature"
  zero_trqEmot1DesPhy/1 -> Bus Creator4/9  "trqEmotDesPhy"
  zero_EMD1_ACT_ReferenceTorqueLimited/1 -> Bus Creator4/8  "EMD_ACT_ReferenceTorqueLimited"
  zero_EMD1_ACT_InverterState/1 -> Bus Creator4/7  "EMD_ACT_InverterState"
  zero_EMD1_ACT_MotorTorque/1 -> Bus Creator4/6  "EMD_ACT_MotorTorque"
  zero_EMD1_ACT_MotorSpeed/1 -> Bus Creator4/5  "EMD_ACT_MotorSpeed"
  zero_EMD1_ACT_DcLinkPower/1 -> Bus Creator4/4  "EMD_ACT_DcLinkPower"
  zero_EMD1_ACT_MaximumAvailableTorque/1 -> Bus Creator4/3  "EMD_ACT_MaximumAvailableTorque"
  zero_EMD1_ACT_DigitalInput1/1 -> Bus Creator4/2  "EMD_ACT_DigitalInput1"
  zero_EMD1_ACT_DcLinkVoltage/1 -> Bus Creator4/1  "EMD1_ACT_DcLinkVoltage"
  Bus Creator4/1 -> Out1/1  "awr1B"

== system Energy_converter_Electrical_to_Mechanical/AWR_DriveEmot/AWR1_4/ZeroWhenNotReady2 ==
  Bus Creator4 : BusCreator  Inputs=11
  zero_EMD4_ACT_DcLinkPower : Constant  Value=0
  zero_EMD4_ACT_DcLinkVoltage : Constant  Value=0
  zero_EMD4_ACT_DigitalInput1 : Constant  Value=0
  zero_EMD4_ACT_InverterState : Constant  Value=0
  zero_EMD4_ACT_MaxJunctionTemperature : Constant  Value=0
  zero_EMD4_ACT_MaximumAvailableTorque : Constant  Value=0
  zero_EMD4_ACT_MotorSpeed : Constant  Value=0
  zero_EMD4_ACT_MotorTemperature : Constant  Value=0
  zero_EMD4_ACT_MotorTorque : Constant  Value=0
  zero_EMD4_ACT_ReferenceTorqueLimited : Constant  Value=0
  zero_trqEmot1DesPhy : Constant  Value=0
  Out1 : Outport
  wires:
  Bus Creator4/1 -> Out1/1  "awr1B"
  zero_EMD4_ACT_DcLinkVoltage/1 -> Bus Creator4/1  "EMD4_ACT_DcLinkVoltage"
  zero_EMD4_ACT_DigitalInput1/1 -> Bus Creator4/2  "EMD_ACT_DigitalInput1"
  zero_EMD4_ACT_MaximumAvailableTorque/1 -> Bus Creator4/3  "EMD_ACT_MaximumAvailableTorque"
  zero_EMD4_ACT_DcLinkPower/1 -> Bus Creator4/4  "EMD_ACT_DcLinkPower"
  zero_EMD4_ACT_MotorSpeed/1 -> Bus Creator4/5  "EMD_ACT_MotorSpeed"
  zero_EMD4_ACT_MotorTorque/1 -> Bus Creator4/6  "EMD_ACT_MotorTorque"
  zero_EMD4_ACT_InverterState/1 -> Bus Creator4/7  "EMD_ACT_InverterState"
  zero_EMD4_ACT_ReferenceTorqueLimited/1 -> Bus Creator4/8  "EMD_ACT_ReferenceTorqueLimited"
  zero_trqEmot1DesPhy/1 -> Bus Creator4/9  "trqEmotDesPhy"
  zero_EMD4_ACT_MaxJunctionTemperature/1 -> Bus Creator4/10  "EMD_ACT_MaxJunctionTemperature"
  zero_EMD4_ACT_MotorTemperature/1 -> Bus Creator4/11  "EMD_ACT_MotorTemperature"

== system Energy_converter_Electrical_to_Mechanical/AWR_DriveEmot/AWR2_3/ZeroWhenNotReady1 ==
  Bus Creator4 : BusCreator  Inputs=11
  zero_EMD1_ACT_DcLinkPower : Constant  Value=0
  zero_EMD1_ACT_DigitalInput1 : Constant  Value=0
  zero_EMD1_ACT_InverterState : Constant  Value=0
  zero_EMD1_ACT_MaxJunctionTemperature : Constant  Value=0
  zero_EMD1_ACT_MaximumAvailableTorque : Constant  Value=0
  zero_EMD1_ACT_MotorSpeed : Constant  Value=0
  zero_EMD1_ACT_MotorTemperature : Constant  Value=0
  zero_EMD1_ACT_MotorTorque : Constant  Value=0
  zero_EMD1_ACT_ReferenceTorqueLimited : Constant  Value=0
  zero_EMD2_ACT_DcLinkVoltage : Constant  Value=0
  zero_trqEmot1DesPhy : Constant  Value=0
  Out1 : Outport
  wires:
  Bus Creator4/1 -> Out1/1  "awr2B"
  zero_EMD2_ACT_DcLinkVoltage/1 -> Bus Creator4/1  "EMD2_ACT_DcLinkVoltage"
  zero_EMD1_ACT_DigitalInput1/1 -> Bus Creator4/2  "EMD_ACT_DigitalInput1"
  zero_EMD1_ACT_MaximumAvailableTorque/1 -> Bus Creator4/3  "EMD_ACT_MaximumAvailableTorque"
  zero_EMD1_ACT_DcLinkPower/1 -> Bus Creator4/4  "EMD_ACT_DcLinkPower"
  zero_EMD1_ACT_MotorSpeed/1 -> Bus Creator4/5  "EMD_ACT_MotorSpeed"
  zero_EMD1_ACT_MotorTorque/1 -> Bus Creator4/6  "EMD_ACT_MotorTorque"
  zero_EMD1_ACT_InverterState/1 -> Bus Creator4/7  "EMD_ACT_InverterState"
  zero_EMD1_ACT_ReferenceTorqueLimited/1 -> Bus Creator4/8  "EMD_ACT_ReferenceTorqueLimited"
  zero_trqEmot1DesPhy/1 -> Bus Creator4/9  "trqEmotDesPhy"
  zero_EMD1_ACT_MaxJunctionTemperature/1 -> Bus Creator4/10  "EMD_ACT_MaxJunctionTemperature"
  zero_EMD1_ACT_MotorTemperature/1 -> Bus Creator4/11  "EMD_ACT_MotorTemperature"

== system Energy_converter_Electrical_to_Mechanical/AWR_DriveEmot/AWR2_3/ZeroWhenNotReady2 ==
  Bus Creator4 : BusCreator  Inputs=11
  zero_EMD3_ACT_DcLinkVoltage : Constant  Value=0
  zero_EMD4_ACT_DcLinkPower : Constant  Value=0
  zero_EMD4_ACT_DigitalInput1 : Constant  Value=0
  zero_EMD4_ACT_InverterState : Constant  Value=0
  zero_EMD4_ACT_MaxJunctionTemperature : Constant  Value=0
  zero_EMD4_ACT_MaximumAvailableTorque : Constant  Value=0
  zero_EMD4_ACT_MotorSpeed : Constant  Value=0
  zero_EMD4_ACT_MotorTemperature : Constant  Value=0
  zero_EMD4_ACT_MotorTorque : Constant  Value=0
  zero_EMD4_ACT_ReferenceTorqueLimited : Constant  Value=0
  zero_trqEmot1DesPhy : Constant  Value=0
  Out1 : Outport
  wires:
  zero_EMD4_ACT_MotorTemperature/1 -> Bus Creator4/11  "EMD_ACT_MotorTemperature"
  zero_EMD4_ACT_MaxJunctionTemperature/1 -> Bus Creator4/10  "EMD_ACT_MaxJunctionTemperature"
  zero_trqEmot1DesPhy/1 -> Bus Creator4/9  "trqEmotDesPhy"
  zero_EMD4_ACT_ReferenceTorqueLimited/1 -> Bus Creator4/8  "EMD_ACT_ReferenceTorqueLimited"
  zero_EMD4_ACT_InverterState/1 -> Bus Creator4/7  "EMD_ACT_InverterState"
  zero_EMD4_ACT_MotorTorque/1 -> Bus Creator4/6  "EMD_ACT_MotorTorque"
  zero_EMD4_ACT_MotorSpeed/1 -> Bus Creator4/5  "EMD_ACT_MotorSpeed"
  zero_EMD4_ACT_DcLinkPower/1 -> Bus Creator4/4  "EMD_ACT_DcLinkPower"
  zero_EMD4_ACT_MaximumAvailableTorque/1 -> Bus Creator4/3  "EMD_ACT_MaximumAvailableTorque"
  zero_EMD4_ACT_DigitalInput1/1 -> Bus Creator4/2  "EMD_ACT_DigitalInput1"
  zero_EMD3_ACT_DcLinkVoltage/1 -> Bus Creator4/1  "EMD3_ACT_DcLinkVoltage"
  Bus Creator4/1 -> Out1/1  "awr3B"

== system Energy_converter_Electrical_to_Mechanical/AWR_DriveEmot/EMD1_CMD_Command/Compare To Constant ==
  u : Inport
  Compare : RelationalOperator  Operator===  OutDataTypeStr=boolean  InputSameDT=on
  Constant : Constant  DisableCoverage=on  Value=const  OutDataTypeStr=Inherit: Inherit via back propagation
  y : Outport
  wires:
  u/1 -> Compare/1
  Constant/1 -> Compare/2
  Compare/1 -> y/1

== system Energy_converter_Electrical_to_Mechanical/AWR_DriveEmot/EMD1_CMD_Command/Compare To Constant1 ==
  u : Inport
  Compare : RelationalOperator  Operator===  OutDataTypeStr=boolean  InputSameDT=on
  Constant : Constant  DisableCoverage=on  Value=const  OutDataTypeStr=Inherit: Inherit via back propagation
  y : Outport
  wires:
  u/1 -> Compare/1
  Constant/1 -> Compare/2
  Compare/1 -> y/1

== system Energy_converter_Electrical_to_Mechanical/AWR_DriveEmot/EMD1_CMD_Command1/Compare To Constant ==
  u : Inport
  Compare : RelationalOperator  Operator===  OutDataTypeStr=boolean  InputSameDT=on
  Constant : Constant  DisableCoverage=on  Value=const  OutDataTypeStr=Inherit: Inherit via back propagation
  y : Outport
  wires:
  u/1 -> Compare/1
  Constant/1 -> Compare/2
  Compare/1 -> y/1

== system Energy_converter_Electrical_to_Mechanical/AWR_DriveEmot/EMD1_CMD_Command1/Compare To Constant1 ==
  u : Inport
  Compare : RelationalOperator  Operator===  OutDataTypeStr=boolean  InputSameDT=on
  Constant : Constant  DisableCoverage=on  Value=const  OutDataTypeStr=Inherit: Inherit via back propagation
  y : Outport
  wires:
  u/1 -> Compare/1
  Constant/1 -> Compare/2
  Compare/1 -> y/1

== system Energy_converter_Electrical_to_Mechanical/AWR_DriveEmot/EMD1_CMD_Command2/Compare To Constant ==
  u : Inport
  Compare : RelationalOperator  Operator===  OutDataTypeStr=boolean  InputSameDT=on
  Constant : Constant  DisableCoverage=on  Value=const  OutDataTypeStr=Inherit: Inherit via back propagation
  y : Outport
  wires:
  u/1 -> Compare/1
  Constant/1 -> Compare/2
  Compare/1 -> y/1

== system Energy_converter_Electrical_to_Mechanical/AWR_DriveEmot/EMD1_CMD_Command2/Compare To Constant1 ==
  u : Inport
  Compare : RelationalOperator  Operator===  OutDataTypeStr=boolean  InputSameDT=on
  Constant : Constant  DisableCoverage=on  Value=const  OutDataTypeStr=Inherit: Inherit via back propagation
  y : Outport
  wires:
  u/1 -> Compare/1
  Constant/1 -> Compare/2
  Compare/1 -> y/1

== system Energy_converter_Electrical_to_Mechanical/AWR_DriveEmot/EMD1_CMD_Command3/Compare To Constant ==
  u : Inport
  Compare : RelationalOperator  Operator===  OutDataTypeStr=boolean  InputSameDT=on
  Constant : Constant  DisableCoverage=on  Value=const  OutDataTypeStr=Inherit: Inherit via back propagation
  y : Outport
  wires:
  u/1 -> Compare/1
  Constant/1 -> Compare/2
  Compare/1 -> y/1

== system Energy_converter_Electrical_to_Mechanical/AWR_DriveEmot/EMD1_CMD_Command3/Compare To Constant1 ==
  u : Inport
  Compare : RelationalOperator  Operator===  OutDataTypeStr=boolean  InputSameDT=on
  Constant : Constant  DisableCoverage=on  Value=const  OutDataTypeStr=Inherit: Inherit via back propagation
  y : Outport
  wires:
  u/1 -> Compare/1
  Constant/1 -> Compare/2
  Compare/1 -> y/1

== system Energy_converter_Electrical_to_Mechanical/AWR_DriveEmot/SummarizeEmotorValuesForVehicle/Avoid_Div_by_zero ==
  U : Inport
  Constant : Constant  Value=10^-6
  Math Function : Math  Operator=reciprocal  SaturateOnIntegerOverflow=on
  Switch : Switch  Criteria=u2 > Threshold
  1/U : Outport
  wires:
  U/1 -> Math Function/1, Switch/2
  Constant/1 -> Switch/3
  Math Function/1 -> Switch/1
  Switch/1 -> 1/U/1

== system Energy_converter_Electrical_to_Mechanical/AWR_DriveEmot_Gen2/AWR 1 TX/Nm_to_percent ==
  Nm_Torque : Inport
  Reference_Torque : Inport  Port=2
  Constant : Constant  Value=100
  Divide1 : Product  Inputs=*/
  Product1 : Product  RndMeth=Zero
  Torque_Percentage : Outport
  wires:
  Nm_Torque/1 -> Divide1/1  "Nm_Torque"
  Product1/1 -> Torque_Percentage/1  "Torque_Percentage"
  Reference_Torque/1 -> Divide1/2  "Reference_Torque"
  Divide1/1 -> Product1/1
  Constant/1 -> Product1/2

== system Energy_converter_Electrical_to_Mechanical/AWR_DriveEmot_Gen2/AWR 1 TX/Nm_to_percent1 ==
  Nm_Torque : Inport
  Reference_Torque : Inport  Port=2
  Constant : Constant  Value=100
  Divide1 : Product  Inputs=*/
  Product1 : Product  RndMeth=Zero
  Torque_Percentage : Outport
  wires:
  Constant/1 -> Product1/2
  Divide1/1 -> Product1/1
  Reference_Torque/1 -> Divide1/2  "Reference_Torque"
  Product1/1 -> Torque_Percentage/1  "Torque_Percentage"
  Nm_Torque/1 -> Divide1/1  "Nm_Torque"

== system Energy_converter_Electrical_to_Mechanical/AWR_DriveEmot_Gen2/AWR 1 TX/Nm_to_percent2 ==
  Nm_Torque : Inport
  Reference_Torque : Inport  Port=2
  Constant : Constant  Value=100
  Divide1 : Product  Inputs=*/
  Product1 : Product  RndMeth=Zero
  Torque_Percentage : Outport
  wires:
  Nm_Torque/1 -> Divide1/1  "Nm_Torque"
  Product1/1 -> Torque_Percentage/1  "Torque_Percentage"
  Reference_Torque/1 -> Divide1/2  "Reference_Torque"
  Divide1/1 -> Product1/1
  Constant/1 -> Product1/2

== system Energy_converter_Electrical_to_Mechanical/AWR_DriveEmot_Gen2/AWR 2 TX/Nm_to_percent ==
  Nm_Torque : Inport
  Reference_Torque : Inport  Port=2
  Constant : Constant  Value=100
  Divide1 : Product  Inputs=*/
  Product1 : Product  RndMeth=Zero
  Torque_Percentage : Outport
  wires:
  Nm_Torque/1 -> Divide1/1  "Nm_Torque"
  Product1/1 -> Torque_Percentage/1  "Torque_Percentage"
  Reference_Torque/1 -> Divide1/2  "Reference_Torque"
  Divide1/1 -> Product1/1
  Constant/1 -> Product1/2

== system Energy_converter_Electrical_to_Mechanical/AWR_DriveEmot_Gen2/AWR 2 TX/Nm_to_percent1 ==
  Nm_Torque : Inport
  Reference_Torque : Inport  Port=2
  Constant : Constant  Value=100
  Divide1 : Product  Inputs=*/
  Product1 : Product  RndMeth=Zero
  Torque_Percentage : Outport
  wires:
  Constant/1 -> Product1/2
  Divide1/1 -> Product1/1
  Reference_Torque/1 -> Divide1/2  "Reference_Torque"
  Product1/1 -> Torque_Percentage/1  "Torque_Percentage"
  Nm_Torque/1 -> Divide1/1  "Nm_Torque"

== system Energy_converter_Electrical_to_Mechanical/AWR_DriveEmot_Gen2/AWR 2 TX/Nm_to_percent2 ==
  Nm_Torque : Inport
  Reference_Torque : Inport  Port=2
  Constant : Constant  Value=100
  Divide1 : Product  Inputs=*/
  Product1 : Product  RndMeth=Zero
  Torque_Percentage : Outport
  wires:
  Nm_Torque/1 -> Divide1/1  "Nm_Torque"
  Product1/1 -> Torque_Percentage/1  "Torque_Percentage"
  Reference_Torque/1 -> Divide1/2  "Reference_Torque"
  Divide1/1 -> Product1/1
  Constant/1 -> Product1/2

== system Energy_converter_Electrical_to_Mechanical/AWR_DriveEmot_Gen2/AWR 3 TX/Nm_to_percent ==
  Nm_Torque : Inport
  Reference_Torque : Inport  Port=2
  Constant : Constant  Value=100
  Divide1 : Product  Inputs=*/
  Product1 : Product  RndMeth=Zero
  Torque_Percentage : Outport
  wires:
  Constant/1 -> Product1/2
  Divide1/1 -> Product1/1
  Reference_Torque/1 -> Divide1/2  "Reference_Torque"
  Product1/1 -> Torque_Percentage/1  "Torque_Percentage"
  Nm_Torque/1 -> Divide1/1  "Nm_Torque"

== system Energy_converter_Electrical_to_Mechanical/AWR_DriveEmot_Gen2/AWR 3 TX/Nm_to_percent1 ==
  Nm_Torque : Inport
  Reference_Torque : Inport  Port=2
  Constant : Constant  Value=100
  Divide1 : Product  Inputs=*/
  Product1 : Product  RndMeth=Zero
  Torque_Percentage : Outport
  wires:
  Nm_Torque/1 -> Divide1/1  "Nm_Torque"
  Product1/1 -> Torque_Percentage/1  "Torque_Percentage"
  Reference_Torque/1 -> Divide1/2  "Reference_Torque"
  Divide1/1 -> Product1/1
  Constant/1 -> Product1/2

== system Energy_converter_Electrical_to_Mechanical/AWR_DriveEmot_Gen2/AWR 3 TX/Nm_to_percent2 ==
  Nm_Torque : Inport
  Reference_Torque : Inport  Port=2
  Constant : Constant  Value=100
  Divide1 : Product  Inputs=*/
  Product1 : Product  RndMeth=Zero
  Torque_Percentage : Outport
  wires:
  Constant/1 -> Product1/2
  Divide1/1 -> Product1/1
  Reference_Torque/1 -> Divide1/2  "Reference_Torque"
  Product1/1 -> Torque_Percentage/1  "Torque_Percentage"
  Nm_Torque/1 -> Divide1/1  "Nm_Torque"

== system Energy_converter_Electrical_to_Mechanical/AWR_DriveEmot_Gen2/AWR 4 TX/Nm_to_percent ==
  Nm_Torque : Inport
  Reference_Torque : Inport  Port=2
  Constant : Constant  Value=100
  Divide1 : Product  Inputs=*/
  Product1 : Product  RndMeth=Zero
  Torque_Percentage : Outport
  wires:
  Nm_Torque/1 -> Divide1/1  "Nm_Torque"
  Product1/1 -> Torque_Percentage/1  "Torque_Percentage"
  Reference_Torque/1 -> Divide1/2  "Reference_Torque"
  Divide1/1 -> Product1/1
  Constant/1 -> Product1/2

== system Energy_converter_Electrical_to_Mechanical/AWR_DriveEmot_Gen2/AWR 4 TX/Nm_to_percent1 ==
  Nm_Torque : Inport
  Reference_Torque : Inport  Port=2
  Constant : Constant  Value=100
  Divide1 : Product  Inputs=*/
  Product1 : Product  RndMeth=Zero
  Torque_Percentage : Outport
  wires:
  Constant/1 -> Product1/2
  Divide1/1 -> Product1/1
  Reference_Torque/1 -> Divide1/2  "Reference_Torque"
  Product1/1 -> Torque_Percentage/1  "Torque_Percentage"
  Nm_Torque/1 -> Divide1/1  "Nm_Torque"

== system Energy_converter_Electrical_to_Mechanical/AWR_DriveEmot_Gen2/AWR 4 TX/Nm_to_percent2 ==
  Nm_Torque : Inport
  Reference_Torque : Inport  Port=2
  Constant : Constant  Value=100
  Divide1 : Product  Inputs=*/
  Product1 : Product  RndMeth=Zero
  Torque_Percentage : Outport
  wires:
  Nm_Torque/1 -> Divide1/1  "Nm_Torque"
  Product1/1 -> Torque_Percentage/1  "Torque_Percentage"
  Reference_Torque/1 -> Divide1/2  "Reference_Torque"
  Divide1/1 -> Product1/1
  Constant/1 -> Product1/2

== system Energy_converter_Electrical_to_Mechanical/AWR_DriveEmot_Gen2/AWR1_4/ZeroWhenNotReady1 ==
  Bus Creator4 : BusCreator  Inputs=11
  zero_EMD1_ACT_DcLinkPower : Constant  Value=0
  zero_EMD1_ACT_DcLinkVoltage : Constant  Value=0
  zero_EMD1_ACT_DigitalInput1 : Constant  Value=0
  zero_EMD1_ACT_InverterState : Constant  Value=0
  zero_EMD1_ACT_MaxJunctionTemperature : Constant  Value=0
  zero_EMD1_ACT_MaximumAvailableTorque : Constant  Value=0
  zero_EMD1_ACT_MotorSpeed : Constant  Value=0
  zero_EMD1_ACT_MotorTemperature : Constant  Value=0
  zero_EMD1_ACT_MotorTorque : Constant  Value=0
  zero_EMD1_ACT_ReferenceTorqueLimited : Constant  Value=0
  zero_trqEmot1DesPhy : Constant  Value=0
  Out1 : Outport
  wires:
  Bus Creator4/1 -> Out1/1  "awr1B"
  zero_EMD1_ACT_DcLinkVoltage/1 -> Bus Creator4/1  "EMD1_ACT_DcLinkVoltage"
  zero_EMD1_ACT_DigitalInput1/1 -> Bus Creator4/2  "EMD_ACT_DigitalInput1"
  zero_EMD1_ACT_MaximumAvailableTorque/1 -> Bus Creator4/3  "EMD_ACT_MaximumAvailableTorque"
  zero_EMD1_ACT_DcLinkPower/1 -> Bus Creator4/4  "EMD_ACT_DcLinkPower"
  zero_EMD1_ACT_MotorSpeed/1 -> Bus Creator4/5  "EMD_ACT_MotorSpeed"
  zero_EMD1_ACT_MotorTorque/1 -> Bus Creator4/6  "EMD_ACT_MotorTorque"
  zero_EMD1_ACT_InverterState/1 -> Bus Creator4/7  "EMD_ACT_InverterState"
  zero_EMD1_ACT_ReferenceTorqueLimited/1 -> Bus Creator4/8  "EMD_ACT_ReferenceTorqueLimited"
  zero_trqEmot1DesPhy/1 -> Bus Creator4/9  "trqEmotDesPhy"
  zero_EMD1_ACT_MaxJunctionTemperature/1 -> Bus Creator4/10  "EMD_ACT_MaxJunctionTemperature"
  zero_EMD1_ACT_MotorTemperature/1 -> Bus Creator4/11  "EMD_ACT_MotorTemperature"

== system Energy_converter_Electrical_to_Mechanical/AWR_DriveEmot_Gen2/AWR1_4/ZeroWhenNotReady2 ==
  Bus Creator4 : BusCreator  Inputs=11
  zero_EMD4_ACT_DcLinkPower : Constant  Value=0
  zero_EMD4_ACT_DcLinkVoltage : Constant  Value=0
  zero_EMD4_ACT_DigitalInput1 : Constant  Value=0
  zero_EMD4_ACT_InverterState : Constant  Value=0
  zero_EMD4_ACT_MaxJunctionTemperature : Constant  Value=0
  zero_EMD4_ACT_MaximumAvailableTorque : Constant  Value=0
  zero_EMD4_ACT_MotorSpeed : Constant  Value=0
  zero_EMD4_ACT_MotorTemperature : Constant  Value=0
  zero_EMD4_ACT_MotorTorque : Constant  Value=0
  zero_EMD4_ACT_ReferenceTorqueLimited : Constant  Value=0
  zero_trqEmot1DesPhy : Constant  Value=0
  Out1 : Outport
  wires:
  zero_EMD4_ACT_MotorTemperature/1 -> Bus Creator4/11  "EMD_ACT_MotorTemperature"
  zero_EMD4_ACT_MaxJunctionTemperature/1 -> Bus Creator4/10  "EMD_ACT_MaxJunctionTemperature"
  zero_trqEmot1DesPhy/1 -> Bus Creator4/9  "trqEmotDesPhy"
  zero_EMD4_ACT_ReferenceTorqueLimited/1 -> Bus Creator4/8  "EMD_ACT_ReferenceTorqueLimited"
  zero_EMD4_ACT_InverterState/1 -> Bus Creator4/7  "EMD_ACT_InverterState"
  zero_EMD4_ACT_MotorTorque/1 -> Bus Creator4/6  "EMD_ACT_MotorTorque"
  zero_EMD4_ACT_MotorSpeed/1 -> Bus Creator4/5  "EMD_ACT_MotorSpeed"
  zero_EMD4_ACT_DcLinkPower/1 -> Bus Creator4/4  "EMD_ACT_DcLinkPower"
  zero_EMD4_ACT_MaximumAvailableTorque/1 -> Bus Creator4/3  "EMD_ACT_MaximumAvailableTorque"
  zero_EMD4_ACT_DigitalInput1/1 -> Bus Creator4/2  "EMD_ACT_DigitalInput1"
  zero_EMD4_ACT_DcLinkVoltage/1 -> Bus Creator4/1  "EMD4_ACT_DcLinkVoltage"
  Bus Creator4/1 -> Out1/1  "awr1B"

== system Energy_converter_Electrical_to_Mechanical/AWR_DriveEmot_Gen2/AWR2_3/ZeroWhenNotReady1 ==
  Bus Creator4 : BusCreator  Inputs=11
  zero_EMD1_ACT_DcLinkPower : Constant  Value=0
  zero_EMD1_ACT_DigitalInput1 : Constant  Value=0
  zero_EMD1_ACT_InverterState : Constant  Value=0
  zero_EMD1_ACT_MaxJunctionTemperature : Constant  Value=0
  zero_EMD1_ACT_MaximumAvailableTorque : Constant  Value=0
  zero_EMD1_ACT_MotorSpeed : Constant  Value=0
  zero_EMD1_ACT_MotorTemperature : Constant  Value=0
  zero_EMD1_ACT_MotorTorque : Constant  Value=0
  zero_EMD1_ACT_ReferenceTorqueLimited : Constant  Value=0
  zero_EMD2_ACT_DcLinkVoltage : Constant  Value=0
  zero_trqEmot1DesPhy : Constant  Value=0
  Out1 : Outport
  wires:
  zero_EMD1_ACT_MotorTemperature/1 -> Bus Creator4/11  "EMD_ACT_MotorTemperature"
  zero_EMD1_ACT_MaxJunctionTemperature/1 -> Bus Creator4/10  "EMD_ACT_MaxJunctionTemperature"
  zero_trqEmot1DesPhy/1 -> Bus Creator4/9  "trqEmotDesPhy"
  zero_EMD1_ACT_ReferenceTorqueLimited/1 -> Bus Creator4/8  "EMD_ACT_ReferenceTorqueLimited"
  zero_EMD1_ACT_InverterState/1 -> Bus Creator4/7  "EMD_ACT_InverterState"
  zero_EMD1_ACT_MotorTorque/1 -> Bus Creator4/6  "EMD_ACT_MotorTorque"
  zero_EMD1_ACT_MotorSpeed/1 -> Bus Creator4/5  "EMD_ACT_MotorSpeed"
  zero_EMD1_ACT_DcLinkPower/1 -> Bus Creator4/4  "EMD_ACT_DcLinkPower"
  zero_EMD1_ACT_MaximumAvailableTorque/1 -> Bus Creator4/3  "EMD_ACT_MaximumAvailableTorque"
  zero_EMD1_ACT_DigitalInput1/1 -> Bus Creator4/2  "EMD_ACT_DigitalInput1"
  zero_EMD2_ACT_DcLinkVoltage/1 -> Bus Creator4/1  "EMD2_ACT_DcLinkVoltage"
  Bus Creator4/1 -> Out1/1  "awr2B"
